simulink model "mSFunction_Fanli"  (Simulink 9.1)
settings: Solver=VariableStepAuto  StartTime=0.0  StopTime=10.0  RelTol=1e-3
libraries: simulink x1
settings Model: Creator=McQueen_Zero  LastModifiedBy=McQueen_Zero
settings DataIOCC: SaveFormat=Dataset
settings OptimizationCC: LifeSpan=auto
settings DebuggingCC: UnderspecifiedInitializationDetection=Simplified  MergeDetectMultiDrivingBlocksExec=error  SFUnexpectedBacktrackingDiag=error  SFNoUnconditionalDefaultTransitionDiag=error  SFExecutionAtInitializationDiag=warning
settings HardwareCC: ProdBitPerPointer=64  ProdBitPerSizeT=64  ProdBitPerPtrDiffT=64  ProdLargestAtomicFloat=Float  ProdIntDivRoundTo=Zero  ProdEndianess=LittleEndian  ProdWordSize=64  ProdHWDeviceType=Intel->x86-64 (Windows64)
settings ModelReferenceCC: PropagateSignalLabelsOutOfModel=on
settings CodeAppCC: StateflowObjectComments=off
settings GRTTargetCC: TargetLangStandard=C99 (ISO)  CombineOutputUpdateFcns=on  GRTInterface=off
settings ConfigComp: CovMetricSettings=dwe  CovHtmlReporting=off  CovSaveCumulativeToWorkspaceVar=off  CovSaveSingleToWorkspaceVar=off  CovExternalEMLEnable=on

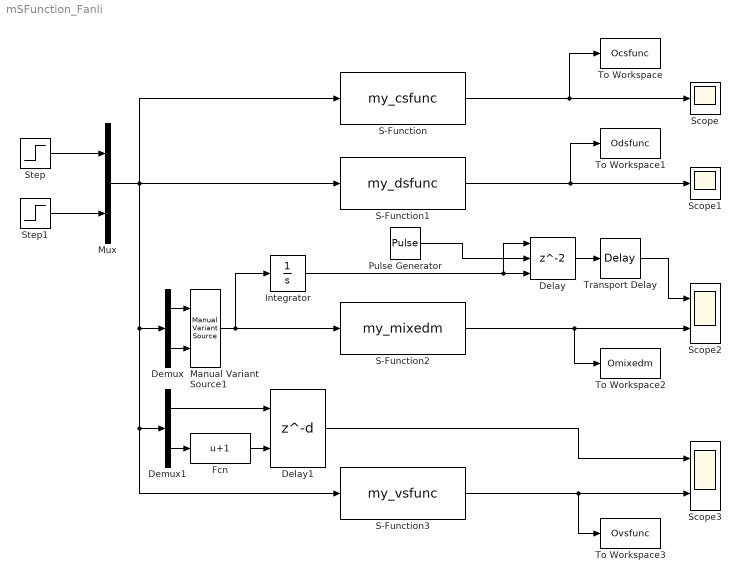
== system mSFunction_Fanli ==
  Delay : Delay  InitialConditionSource=Input port  InitialCondition=1  ExternalReset=Either
      settings: InputPortMap=u0,r5,p4
  Delay1 : Delay  DelayLengthSource=Input port  DelayLength=1  InitialCondition=0
      settings: InputPortMap=u0,p1
  Demux : Demux  Outputs=2
  Demux1 : Demux  Outputs=2
  Fcn : Fcn  Expr=u+1
  Integrator : Integrator  InitialCondition=1
  Manual Variant Source1 : simulink/Signal Routing/Manual Variant Source  NumChoices=2  OverrideUsingVariant=V_1
      settings: SourceProductName=Simulink
  Mux : Mux  Inputs=2
  Pulse Generator : DiscretePulseGenerator  PulseType=Time based  Period=4  PulseWidth=50  PhaseDelay=2
  S-Function : S-Function  FunctionName=my_csfunc  SFunctionDeploymentMode=off  EnableBusSupport=off
  S-Function1 : S-Function  FunctionName=my_dsfunc  SFunctionDeploymentMode=off  EnableBusSupport=off
  S-Function2 : S-Function  FunctionName=my_mixedm  SFunctionDeploymentMode=off  EnableBusSupport=off
  S-Function3 : S-Function  FunctionName=my_vsfunc  SFunctionDeploymentMode=off  EnableBusSupport=off
  Scope : Scope
  Scope1 : Scope
  Scope2 : Scope  NumInputPorts=2
  Scope3 : Scope  NumInputPorts=2
  Step : Step  Time=0  SampleTime=0
  Step1 : Step  Time=0  After=2  SampleTime=0
  To Workspace : ToWorkspace  VariableName=Ocsfunc  SaveFormat=Timeseries  SampleTime=-1
  To Workspace1 : ToWorkspace  VariableName=Odsfunc  SaveFormat=Timeseries  SampleTime=-1
  To Workspace2 : ToWorkspace  VariableName=Omixedm  SaveFormat=Timeseries  SampleTime=-1
  To Workspace3 : ToWorkspace  VariableName=Ovsfunc  SaveFormat=Timeseries  SampleTime=-1
  Transport Delay : TransportDelay  DelayTime=2  InitialOutput=1
  wires:
  Step/1 -> Mux/1
  S-Function3/1 -> To Workspace3/1, Scope3/2
  S-Function2/1 -> To Workspace2/1, Scope2/2
  S-Function/1 -> To Workspace/1, Scope/1
  Step1/1 -> Mux/2
  Demux/1 -> Manual Variant Source1/1
  Demux/2 -> Manual Variant Source1/2
  S-Function1/1 -> To Workspace1/1, Scope1/1
  Integrator/1 -> Delay/1, Delay/3
  Delay/1 -> Transport Delay/1
  Manual Variant Source1/1 -> S-Function2/1, Integrator/1
  Pulse Generator/1 -> Delay/2
  Transport Delay/1 -> Scope2/1
  Mux/1 -> Demux1/1, S-Function3/1, Demux/1, S-Function/1, S-Function1/1
  Demux1/2 -> Fcn/1
  Delay1/1 -> Scope3/1
  Fcn/1 -> Delay1/2
  Demux1/1 -> Delay1/1
